simulink model "systemTest_06_24_14_05_13am"  (R2014a)
settings: Solver=ode45  StartTime=0.0  StopTime=100  RelTol=1e-3
values from neighbouring files (symbols this model uses):
  C = [1 0 0 0 0 0;0 0 1 0 0 0;0 0 0 0 1 0]    [parameters1.m]
  friX1 = 4    [initial_parameters.m]    (also in parameters1.m)
  friX2 = 0.76462    [initial_parameters.m]    (also in parameters1.m)
  friY = 8    [initial_parameters.m]    (also in parameters1.m)
  friZ = 4    [initial_parameters.m]    (also in parameters1.m)
  I = 1/12*m*((2*ry1)^2 + (2*rx1)^2)    (= 25.431685482)    [initial_parameters.m]    (also in parameters1.m = 15)
  inputBound = [minInput maxInput]    [parameters1.m]
  K = [1000 1000 1000 10 10 1 1]    [parameters1.m]
  k1m = 50    [parameters1.m]
  k1x = 100    [parameters1.m]
  k1y = 100    [parameters1.m]
  k2m = 25    [parameters1.m]
  k2x = 60    [parameters1.m]
  k2y = 60    [parameters1.m]
  m = 46.27    [initial_parameters.m]    (also in parameters1.m)
  rx1 = -1.2474    [initial_parameters.m]    (also in parameters1.m = -0.7)
  rx2 = rx1    (= -1.2474)    [initial_parameters.m]    (also in parameters1.m = -0.7)
  ry1 = 12*intom    (= 0.3048)    [initial_parameters.m]    (also in parameters1.m)
  ry2 = -12*intom    (= -0.3048)    [initial_parameters.m]    (also in parameters1.m)
libraries: simulink x6
settings Model: Creator=propagator  LastModifiedBy=propagator

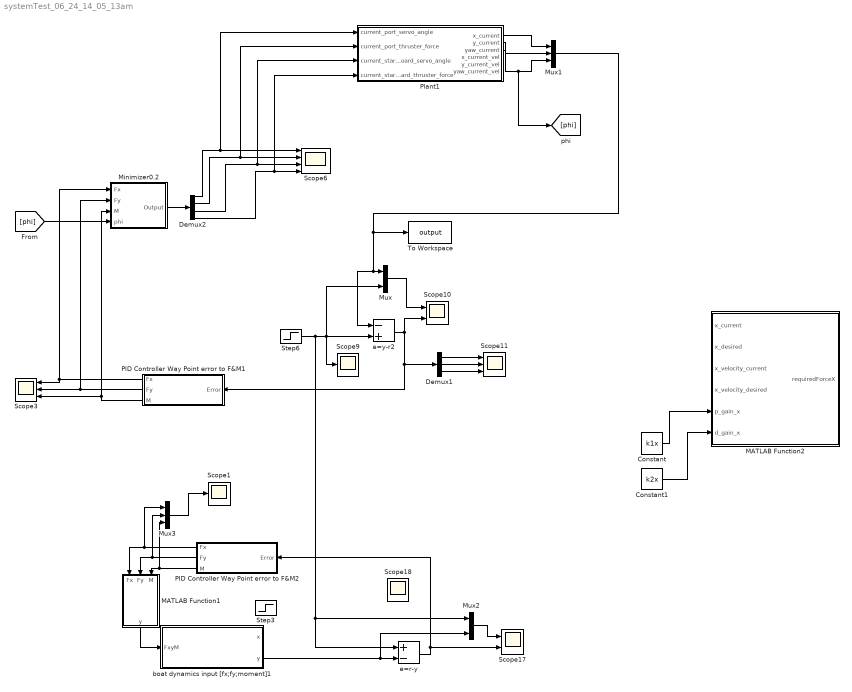
== system systemTest_06_24_14_05_13am ==
  Constant : Constant  Value=k1x
  Constant1 : Constant  Value=k2x
  Demux1 : Demux  Outputs=3
  Demux2 : Demux
  MATLAB Function1 : MATLAB Function  TreatAsAtomicUnit=on
  MATLAB Function2 : MATLAB Function  TreatAsAtomicUnit=on
  Minimizer0.2 : Subsystem  mask{rx1=rx1, rx2=rx2, ry1=ry1, ry2=ry2, C=K, inputBound=inputBound, m=m, I=I}
      mask prompts: C "Performance Gain"; inputBound "Input Bounds"; m "Boat Mass"; I "Boat Inertia"
      mask TypeOptions m: Constant6/Value
      mask TypeOptions I: Constant7/Value
  Mux : Mux  Inputs=2
  Mux1 : Mux  Inputs=3
  Mux2 : Mux  Inputs=2
  Mux3 : Mux  Inputs=3
  PID Controller Way Point error to F&M1 : Subsystem
  PID Controller Way Point error to F&M2 : Subsystem
  Plant1 : Subsystem  mask{rx1=rx1, ry1=ry1, ry2=ry2, M=m, I=I, friX1=friX1, friX2=friX2, friY=friY, friZ=friZ}
      mask TypeOptions rx1: Constant/Value
      mask TypeOptions friX1: Constant1/Value
      mask TypeOptions friX2: Constant8/Value
      mask TypeOptions friY: Constant7/Value
      mask TypeOptions friZ: Constant9/Value
  Scope1 : Scope
      settings: YMin=-0.014  YMax=0  SaveName=ScopeData4
  Scope10 : Scope  NumInputPorts=2
      settings: YMin=0~-0.04  YMax=2~0.025  SaveName=ScopeData9
  Scope11 : Scope  NumInputPorts=3
      settings: YMin=8.65~2.725~-26.6  YMax=8.975~2.925~-25.6  SaveName=ScopeData11
  Scope17 : Scope  NumInputPorts=2
      settings: YMin=0~0  YMax=70~17
  Scope18 : Scope
      settings: SaveName=ScopeData2
  Scope3 : Scope  NumInputPorts=3
      settings: YMin=-1.25~-1~7000  YMax=0.75~1~7000  SaveName=ScopeData3
  Scope6 : Scope  NumInputPorts=4
      settings: YMin=-28~-100~15~0  YMax=-15~0~28~100  SaveName=ScopeData5
  Scope9 : Scope
      settings: SaveName=ScopeData8
  Step3 : Step  Before=[0;0;0]  After=[15;1;1]  SampleTime=0
  Step6 : Step  Before=[0;0;0]  After=[10;0;0]  SampleTime=0
  To Workspace : ToWorkspace  VariableName=output  SaveFormat=Timeseries  SampleTime=-1
  boat dynamics input [fx;fy;moment]1 : Subsystem  mask{M=m, I=I, fw=0, kr=0, C=C}
      mask prompts: M "Mass"; I "Inert"; fw "Water Friction"; kr "Rotational water Friction"; C "Output Matrix"
  e=r-y : Sum  Inputs=+-
  e=y-r2 : Sum  Inputs=-+
  wires:
  Demux2/1 -> Plant1/1(current_port_servo_angle), Scope6/1
  Demux2/2 -> Plant1/2(current_port_thruster_force), Scope6/2
  Demux2/3 -> Plant1/3(current_starboard_servo_angle), Scope6/3
  Demux2/4 -> Plant1/4(current_starboard_thruster_force), Scope6/4
  Minimizer0.2/1(Output) -> Demux2/1
  Step6/1 -> Mux2/1, e=r-y/1, Mux/2, e=y-r2/2, Scope9/1
  e=y-r2/1 -> PID Controller Way Point error to F&M1/1(Error), Demux1/1, Scope10/2
  Mux/1 -> Scope10/1
  PID Controller Way Point error to F&M1/1(Fx) -> Minimizer0.2/1(Fx), Scope3/1
  PID Controller Way Point error to F&M1/2(Fy) -> Scope3/2, Minimizer0.2/2(Fy)
  PID Controller Way Point error to F&M1/3(M) -> Scope3/3, Minimizer0.2/3(M)
  Demux1/3 -> Scope11/3
  Demux1/2 -> Scope11/2
  Demux1/1 -> Scope11/1
  [phi] -> Minimizer0.2/4(phi)
  Plant1/3(yaw_current) -> Mux1/3, [phi]
  Plant1/2(y_current) -> Mux1/2
  Plant1/1(x_current) -> Mux1/1
  Mux1/1 -> e=y-r2/1, Mux/1, To Workspace/1
  e=r-y/1 -> PID Controller Way Point error to F&M2/1(Error), Scope17/2
  PID Controller Way Point error to F&M2/1(Fx) -> Mux3/1, MATLAB Function1/1(Fx)
  MATLAB Function1/1(y) -> boat dynamics input [fx;fy;moment]1/1(FxyM)
  PID Controller Way Point error to F&M2/2(Fy) -> Mux3/2, MATLAB Function1/2(Fy)
  PID Controller Way Point error to F&M2/3(M) -> Mux3/3, MATLAB Function1/3(M)
  boat dynamics input [fx;fy;moment]1/2(y) -> Mux2/2, e=r-y/2
  Mux2/1 -> Scope17/1
  Mux3/1 -> Scope1/1
  Constant1/1 -> MATLAB Function2/6(d_gain_x)
  Constant/1 -> MATLAB Function2/5(p_gain_x)

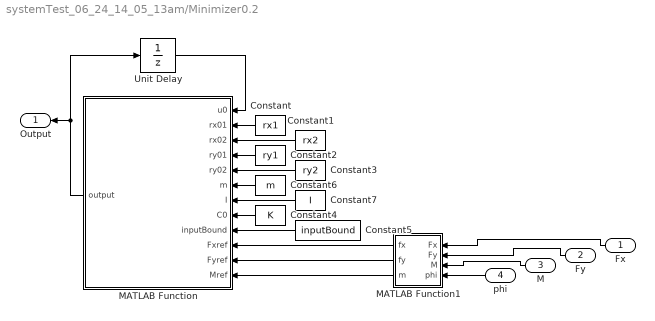
== system systemTest_06_24_14_05_13am/Minimizer0.2 ==
  Fx : Inport
  Fy : Inport  Port=2
  M : Inport  Port=3
  phi : Inport  Port=4
  Constant : Constant  Value=rx1
  Constant1 : Constant  Value=rx2
  Constant2 : Constant  Value=ry1
  Constant3 : Constant  Value=ry2
  Constant4 : Constant  Value=K
  Constant5 : Constant  Value=inputBound
  Constant6 : Constant  Value=m
  Constant7 : Constant  Value=I
  MATLAB Function : MATLAB Function  TreatAsAtomicUnit=on
  MATLAB Function1 : MATLAB Function  TreatAsAtomicUnit=on
  Unit Delay : UnitDelay  InitialCondition=[0;0;0;0]  SampleTime=-1
  Output : Outport
  wires:
  Constant/1 -> MATLAB Function/2(rx01)
  Constant1/1 -> MATLAB Function/3(rx02)
  Constant2/1 -> MATLAB Function/4(ry01)
  Constant4/1 -> MATLAB Function/8(C0)
  Unit Delay/1 -> MATLAB Function/1(u0)
  MATLAB Function/1(output) -> Unit Delay/1, Output/1
  Constant5/1 -> MATLAB Function/9(inputBound)
  Constant3/1 -> MATLAB Function/5(ry02)
  MATLAB Function1/3(m) -> MATLAB Function/12(Mref)
  MATLAB Function1/2(fy) -> MATLAB Function/11(Fyref)
  MATLAB Function1/1(fx) -> MATLAB Function/10(Fxref)
  Fy/1 -> MATLAB Function1/2(Fy)
  Fx/1 -> MATLAB Function1/1(Fx)
  M/1 -> MATLAB Function1/3(M)
  phi/1 -> MATLAB Function1/4(phi)
  Constant6/1 -> MATLAB Function/6(m)
  Constant7/1 -> MATLAB Function/7(I)

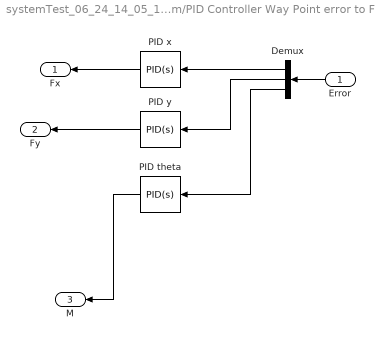
== system systemTest_06_24_14_05_13am/PID Controller Way Point error to F&M1 ==
  Error : Inport
  Demux : Demux  Outputs=3
  PID theta : simulink/Continuous/PID Controller  Controller=PID  TimeDomain=Continuous-time  SampleTime=1  IntegratorMethod=Forward Euler  FilterMethod=Forward Euler  Form=Parallel  P=k1m  I=0  D=k2m  N=3.646824066771  InitialConditionSource=internal  InitialConditionForIntegrator=0  InitialConditionForFilter=0  ExternalReset=none  LimitOutput=off  UpperSaturationLimit=inf  LowerSaturationLimit=-inf  LinearizeAsGain=off  AntiWindupMode=none  Kb=1  TrackingMode=off  Kt=1  PParamMin=[]  PParamMax=[]  IParamMin=[]  IParamMax=[]  DParamMin=[]  DParamMax=[]  NParamMin=[]  NParamMax=[]  KbParamMin=[]  KbParamMax=[]  KtParamMin=[]  KtParamMax=[]  POutMin=[]  POutMax=[]  IOutMin=[]  IOutMax=[]  DOutMin=[]  DOutMax=[]  NOutMin=[]  NOutMax=[]  KbOutMin=[]  KbOutMax=[]  KtOutMin=[]  KtOutMax=[]  IntegratorOutMin=[]  IntegratorOutMax=[]  FilterOutMin=[]  FilterOutMax=[]  SumOutMin=[]  SumOutMax=[]  SumI1OutMin=[]  SumI1OutMax=[]  SumI2OutMin=[]  SumI2OutMax=[]  SumI3OutMin=[]  SumI3OutMax=[]  SumDOutMin=[]  SumDOutMax=[]  SaturationOutMin=[]  SaturationOutMax=[]  IntegratorContinuousStateAttributes=''  IntegratorStateMustResolveToSignalObject=off  IntegratorRTWStateStorageClass=Auto  FilterContinuousStateAttributes=''  FilterStateMustResolveToSignalObject=off  FilterRTWStateStorageClass=Auto
  PID x : simulink/Continuous/PID Controller  Controller=PID  TimeDomain=Continuous-time  SampleTime=1  IntegratorMethod=Forward Euler  FilterMethod=Forward Euler  Form=Parallel  P=k1x  I=0  D=k2x  N=3.646824066771  InitialConditionSource=internal  InitialConditionForIntegrator=0  InitialConditionForFilter=0  ExternalReset=none  LimitOutput=off  UpperSaturationLimit=inf  LowerSaturationLimit=-inf  LinearizeAsGain=off  AntiWindupMode=none  Kb=1  TrackingMode=off  Kt=1  PParamMin=[]  PParamMax=[]  IParamMin=[]  IParamMax=[]  DParamMin=[]  DParamMax=[]  NParamMin=[]  NParamMax=[]  KbParamMin=[]  KbParamMax=[]  KtParamMin=[]  KtParamMax=[]  POutMin=[]  POutMax=[]  IOutMin=[]  IOutMax=[]  DOutMin=[]  DOutMax=[]  NOutMin=[]  NOutMax=[]  KbOutMin=[]  KbOutMax=[]  KtOutMin=[]  KtOutMax=[]  IntegratorOutMin=[]  IntegratorOutMax=[]  FilterOutMin=[]  FilterOutMax=[]  SumOutMin=[]  SumOutMax=[]  SumI1OutMin=[]  SumI1OutMax=[]  SumI2OutMin=[]  SumI2OutMax=[]  SumI3OutMin=[]  SumI3OutMax=[]  SumDOutMin=[]  SumDOutMax=[]  SaturationOutMin=[]  SaturationOutMax=[]  IntegratorContinuousStateAttributes=''  IntegratorStateMustResolveToSignalObject=off  IntegratorRTWStateStorageClass=Auto  FilterContinuousStateAttributes=''  FilterStateMustResolveToSignalObject=off  FilterRTWStateStorageClass=Auto
  PID y : simulink/Continuous/PID Controller  Controller=PID  TimeDomain=Continuous-time  SampleTime=1  IntegratorMethod=Forward Euler  FilterMethod=Forward Euler  Form=Parallel  P=k1y  I=0  D=k2y  N=4  InitialConditionSource=internal  InitialConditionForIntegrator=0  InitialConditionForFilter=0  ExternalReset=none  LimitOutput=off  UpperSaturationLimit=inf  LowerSaturationLimit=-inf  LinearizeAsGain=off  AntiWindupMode=none  Kb=1  TrackingMode=off  Kt=1  PParamMin=[]  PParamMax=[]  IParamMin=[]  IParamMax=[]  DParamMin=[]  DParamMax=[]  NParamMin=[]  NParamMax=[]  KbParamMin=[]  KbParamMax=[]  KtParamMin=[]  KtParamMax=[]  POutMin=[]  POutMax=[]  IOutMin=[]  IOutMax=[]  DOutMin=[]  DOutMax=[]  NOutMin=[]  NOutMax=[]  KbOutMin=[]  KbOutMax=[]  KtOutMin=[]  KtOutMax=[]  IntegratorOutMin=[]  IntegratorOutMax=[]  FilterOutMin=[]  FilterOutMax=[]  SumOutMin=[]  SumOutMax=[]  SumI1OutMin=[]  SumI1OutMax=[]  SumI2OutMin=[]  SumI2OutMax=[]  SumI3OutMin=[]  SumI3OutMax=[]  SumDOutMin=[]  SumDOutMax=[]  SaturationOutMin=[]  SaturationOutMax=[]  IntegratorContinuousStateAttributes=''  IntegratorStateMustResolveToSignalObject=off  IntegratorRTWStateStorageClass=Auto  FilterContinuousStateAttributes=''  FilterStateMustResolveToSignalObject=off  FilterRTWStateStorageClass=Auto
  Fx : Outport
  Fy : Outport  Port=2
  M : Outport  Port=3
  wires:
  Demux/1 -> PID x/1
  Demux/2 -> PID y/1
  Demux/3 -> PID theta/1
  Error/1 -> Demux/1
  PID y/1 -> Fy/1
  PID x/1 -> Fx/1
  PID theta/1 -> M/1

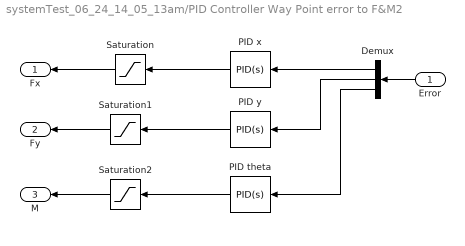
== system systemTest_06_24_14_05_13am/PID Controller Way Point error to F&M2 ==
  Error : Inport
  Demux : Demux  Outputs=3
  PID theta : simulink/Continuous/PID Controller  Controller=PID  TimeDomain=Continuous-time  SampleTime=1  IntegratorMethod=Forward Euler  FilterMethod=Forward Euler  Form=Parallel  P=k1m  I=0  D=k2m  N=3.646824066771  InitialConditionSource=internal  InitialConditionForIntegrator=0  InitialConditionForFilter=0  ExternalReset=none  LimitOutput=off  UpperSaturationLimit=inf  LowerSaturationLimit=-inf  LinearizeAsGain=off  AntiWindupMode=none  Kb=1  TrackingMode=off  Kt=1  PParamMin=[]  PParamMax=[]  IParamMin=[]  IParamMax=[]  DParamMin=[]  DParamMax=[]  NParamMin=[]  NParamMax=[]  KbParamMin=[]  KbParamMax=[]  KtParamMin=[]  KtParamMax=[]  POutMin=[]  POutMax=[]  IOutMin=[]  IOutMax=[]  DOutMin=[]  DOutMax=[]  NOutMin=[]  NOutMax=[]  KbOutMin=[]  KbOutMax=[]  KtOutMin=[]  KtOutMax=[]  IntegratorOutMin=[]  IntegratorOutMax=[]  FilterOutMin=[]  FilterOutMax=[]  SumOutMin=[]  SumOutMax=[]  SumI1OutMin=[]  SumI1OutMax=[]  SumI2OutMin=[]  SumI2OutMax=[]  SumI3OutMin=[]  SumI3OutMax=[]  SumDOutMin=[]  SumDOutMax=[]  SaturationOutMin=[]  SaturationOutMax=[]  IntegratorContinuousStateAttributes=''  IntegratorStateMustResolveToSignalObject=off  IntegratorRTWStateStorageClass=Auto  FilterContinuousStateAttributes=''  FilterStateMustResolveToSignalObject=off  FilterRTWStateStorageClass=Auto
  PID x : simulink/Continuous/PID Controller  Controller=PID  TimeDomain=Continuous-time  SampleTime=1  IntegratorMethod=Forward Euler  FilterMethod=Forward Euler  Form=Parallel  P=k1x  I=0  D=k2x  N=3.646824066771  InitialConditionSource=internal  InitialConditionForIntegrator=0  InitialConditionForFilter=0  ExternalReset=none  LimitOutput=off  UpperSaturationLimit=inf  LowerSaturationLimit=-inf  LinearizeAsGain=off  AntiWindupMode=none  Kb=1  TrackingMode=off  Kt=1  PParamMin=[]  PParamMax=[]  IParamMin=[]  IParamMax=[]  DParamMin=[]  DParamMax=[]  NParamMin=[]  NParamMax=[]  KbParamMin=[]  KbParamMax=[]  KtParamMin=[]  KtParamMax=[]  POutMin=[]  POutMax=[]  IOutMin=[]  IOutMax=[]  DOutMin=[]  DOutMax=[]  NOutMin=[]  NOutMax=[]  KbOutMin=[]  KbOutMax=[]  KtOutMin=[]  KtOutMax=[]  IntegratorOutMin=[]  IntegratorOutMax=[]  FilterOutMin=[]  FilterOutMax=[]  SumOutMin=[]  SumOutMax=[]  SumI1OutMin=[]  SumI1OutMax=[]  SumI2OutMin=[]  SumI2OutMax=[]  SumI3OutMin=[]  SumI3OutMax=[]  SumDOutMin=[]  SumDOutMax=[]  SaturationOutMin=[]  SaturationOutMax=[]  IntegratorContinuousStateAttributes=''  IntegratorStateMustResolveToSignalObject=off  IntegratorRTWStateStorageClass=Auto  FilterContinuousStateAttributes=''  FilterStateMustResolveToSignalObject=off  FilterRTWStateStorageClass=Auto
  PID y : simulink/Continuous/PID Controller  Controller=PID  TimeDomain=Continuous-time  SampleTime=1  IntegratorMethod=Forward Euler  FilterMethod=Forward Euler  Form=Parallel  P=k1y  I=0  D=k2y  N=4  InitialConditionSource=internal  InitialConditionForIntegrator=0  InitialConditionForFilter=0  ExternalReset=none  LimitOutput=off  UpperSaturationLimit=inf  LowerSaturationLimit=-inf  LinearizeAsGain=off  AntiWindupMode=none  Kb=1  TrackingMode=off  Kt=1  PParamMin=[]  PParamMax=[]  IParamMin=[]  IParamMax=[]  DParamMin=[]  DParamMax=[]  NParamMin=[]  NParamMax=[]  KbParamMin=[]  KbParamMax=[]  KtParamMin=[]  KtParamMax=[]  POutMin=[]  POutMax=[]  IOutMin=[]  IOutMax=[]  DOutMin=[]  DOutMax=[]  NOutMin=[]  NOutMax=[]  KbOutMin=[]  KbOutMax=[]  KtOutMin=[]  KtOutMax=[]  IntegratorOutMin=[]  IntegratorOutMax=[]  FilterOutMin=[]  FilterOutMax=[]  SumOutMin=[]  SumOutMax=[]  SumI1OutMin=[]  SumI1OutMax=[]  SumI2OutMin=[]  SumI2OutMax=[]  SumI3OutMin=[]  SumI3OutMax=[]  SumDOutMin=[]  SumDOutMax=[]  SaturationOutMin=[]  SaturationOutMax=[]  IntegratorContinuousStateAttributes=''  IntegratorStateMustResolveToSignalObject=off  IntegratorRTWStateStorageClass=Auto  FilterContinuousStateAttributes=''  FilterStateMustResolveToSignalObject=off  FilterRTWStateStorageClass=Auto
  Saturation : Saturate  UpperLimit=100  LowerLimit=-100
  Saturation1 : Saturate  UpperLimit=100  LowerLimit=-100
  Saturation2 : Saturate  UpperLimit=50  LowerLimit=-50
  Fx : Outport
  Fy : Outport  Port=2
  M : Outport  Port=3
  wires:
  Demux/1 -> PID x/1
  Demux/2 -> PID y/1
  Demux/3 -> PID theta/1
  Error/1 -> Demux/1
  PID x/1 -> Saturation/1
  Saturation/1 -> Fx/1
  PID y/1 -> Saturation1/1
  Saturation1/1 -> Fy/1
  PID theta/1 -> Saturation2/1
  Saturation2/1 -> M/1

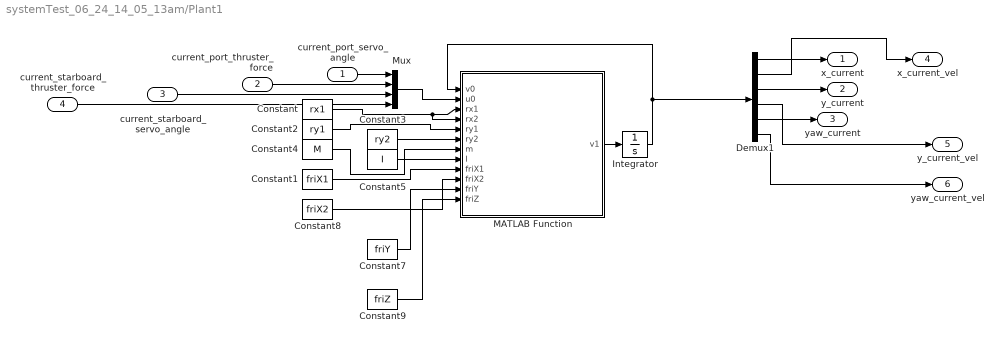
== system systemTest_06_24_14_05_13am/Plant1 ==
  current_port_servo_angle : Inport
  current_port_thruster_force : Inport  Port=2
  current_starboard_servo_angle : Inport  Port=3
  current_starboard_thruster_force : Inport  Port=4
  Constant : Constant  Value=rx1
  Constant1 : Constant  Value=friX1
  Constant2 : Constant  Value=ry1
  Constant3 : Constant  Value=ry2
  Constant4 : Constant  Value=M
  Constant5 : Constant  Value=I
  Constant7 : Constant  Value=friY
  Constant8 : Constant  Value=friX2
  Constant9 : Constant  Value=friZ
  Demux1 : Demux  Outputs=6
  Integrator : Integrator  InitialCondition=[0 0 0 0 0 0]
  MATLAB Function : MATLAB Function  TreatAsAtomicUnit=on
  Mux : Mux
  x_current : Outport
  y_current : Outport  Port=2
  yaw_current : Outport  Port=3
  x_current_vel : Outport  Port=4
  y_current_vel : Outport  Port=5
  yaw_current_vel : Outport  Port=6
  wires:
  Constant/1 -> MATLAB Function/3(rx1), MATLAB Function/4(rx2)
  Constant2/1 -> MATLAB Function/5(ry1)
  Constant3/1 -> MATLAB Function/6(ry2)
  Constant4/1 -> MATLAB Function/7(m)
  Constant5/1 -> MATLAB Function/8(I)
  MATLAB Function/1(v1) -> Integrator/1
  Integrator/1 -> MATLAB Function/1(v0), Demux1/1
  current_port_servo_angle/1 -> Mux/1
  current_port_thruster_force/1 -> Mux/2
  current_starboard_servo_angle/1 -> Mux/3
  current_starboard_thruster_force/1 -> Mux/4
  Mux/1 -> MATLAB Function/2(u0)
  Constant1/1 -> MATLAB Function/9(friX1)
  Constant7/1 -> MATLAB Function/11(friY)
  Constant9/1 -> MATLAB Function/12(friZ)
  Constant8/1 -> MATLAB Function/10(friX2)
  Demux1/5 -> yaw_current/1
  Demux1/3 -> y_current/1
  Demux1/1 -> x_current/1
  Demux1/2 -> x_current_vel/1
  Demux1/4 -> y_current_vel/1
  Demux1/6 -> yaw_current_vel/1

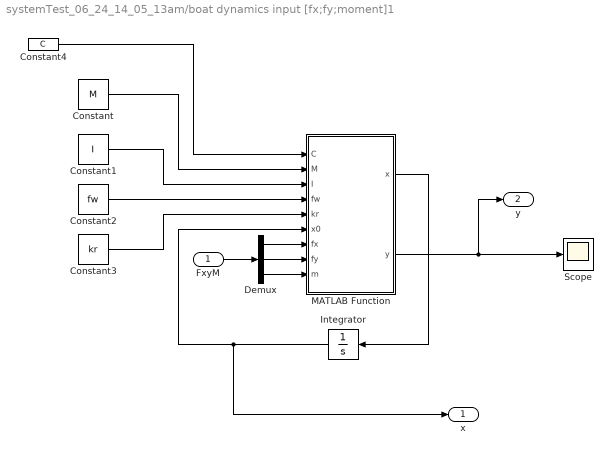
== system systemTest_06_24_14_05_13am/boat dynamics input [fx;fy;moment]1 ==
  FxyM : Inport
  Constant : Constant  Value=M
  Constant1 : Constant  Value=I
  Constant2 : Constant  Value=fw
  Constant3 : Constant  Value=kr
  Constant4 : Constant  Value=C
  Demux : Demux  Outputs=3
  Integrator : Integrator  InitialCondition=[0 0 0 0 0 0]
  MATLAB Function : MATLAB Function  TreatAsAtomicUnit=on
  Scope : Scope
  x : Outport
  y : Outport  Port=2
  wires:
  MATLAB Function/2(y) -> Scope/1, y/1
  Integrator/1 -> x/1, MATLAB Function/6(x0)
  Constant/1 -> MATLAB Function/2(M)
  Constant1/1 -> MATLAB Function/3(I)
  Constant2/1 -> MATLAB Function/4(fw)
  Constant3/1 -> MATLAB Function/5(kr)
  Constant4/1 -> MATLAB Function/1(C)
  MATLAB Function/1(x) -> Integrator/1
  FxyM/1 -> Demux/1
  Demux/1 -> MATLAB Function/7(fx)
  Demux/2 -> MATLAB Function/8(fy)
  Demux/3 -> MATLAB Function/9(m)

== matlab function systemTest_06_24_14_05_13am/MATLAB Function2 ==
  data: x_current input; requiredForceX output; x_desired input; x_velocity_current input; x_velocity_desired input; p_gain_x input; d_gain_x input
function requiredForceX = fcn(x_current,x_desired,x_velocity_current,x_velocity_desired, p_gain_x, d_gain_x)
%#codegen


requiredForceX = p_gain_x * (x_desired - x_current) + d_gain_x * (x_velocity_desired - x_velocity_current);
end

== matlab function systemTest_06_24_14_05_13am/Plant1/MATLAB Function ==
  data: v0 input; v1 output; u0 input; rx1 input; rx2 input; ry1 input; ry2 input; m input; I input; friX1 input; friX2 input; friY input; friZ input

function v1   = boatDynamics(v0, u0, rx1, rx2, ry1, ry2, m, I, friX1,friX2, friY, friZ)

    % %%%%%%%%%%%%%%%%%%%%%%%%%%%%%%%%%%%%%%%%%%%% %
    %    v = [x...          %    u = [theta1...    %
    %        x_dot...       %        f1...         %
    %        y...           %        theta2...     %
    %        y_dot...       %        f2]           %
    %        theta...       %                      %
    %        theta_dot];    %                      %
    % %%%%%%%%%%%%%%%%%%%%%%%%%%%%%%%%%%%%%%%%%%%% %
    
    v11 = v0(2);
    v12 = u0(2)/m*cosd(u0(1)+v0(5)) + u0(4)/m*cosd(u0(3)+v0(5)) - (friX1*v0(2)*(cosd(v0(5))+sind(v0(5))) - friX2*(v0(2)*(cosd(v0(5))+sind(v0(5))))^2);
    v13 = v0(4);
    v14 = u0(2)/m*sind(u0(1)+v0(5)) + u0(4)/m*sind(u0(3)+v0(5)) - friY*v0(4)*(-sind(v0(5))+cosd(v0(5)));
    v15 = v0(6);
    v16 = -rx1/I*u0(2)*sind(u0(1)) + ry1/I*u0(2)*cosd(u0(1)) - rx2/I*u0(4)*sind(u0(3)) + ry2/I*u0(4)*cosd(u0(3)) - friZ*v0(6);
   
    v1 = [v11;v12;v13;v14;v15;v16];
    
end

== matlab function systemTest_06_24_14_05_13am/Minimizer0.2/MATLAB Function ==
  data: u0 input; output output; rx01 input; rx02 input; ry01 input; ry02 input; m input; I input; C0 input; inputBound input; Fxref input; Fyref input; Mref input
function output = Minimizer(u0, rx01, rx02, ry01, ry02, m, I, C0, inputBound, Fxref, Fyref, Mref)

rx1 = rx01; rx2 = rx02;
ry1 = ry01; ry2 = ry02;

C = C0;

%Fxref = Fx; Fyref = Fy; Mref  = M;

gridNum = 10;

grid = boundGrid(inputBound, gridNum, rx1,ry1);

u1 = getMinFromGrid(grid, u0, Fxref, Fyref, Mref, rx1, rx2, ry1, ry2, C, m, I);

% u1 = u0;

% %     for k = 1:20
% %         h = getDirection(u1, u0, Fxref, Fyref, Mref, rx1, rx2, ry1, ry2, C);
% %         alpha = getStepSize(u1, u0, h, Fxref, Fyref, Mref, rx1, rx2, ry1, ry2, C);
% %         u1 = u1 + alpha*h;
% %         u1 = checkInputBound(u1,inputBound);
% %     end
    
    output = u1;

end

function output = getMinFromGrid(grid, preinput, Fxref, Fyref, Mref, rx1, rx2, ry1, ry2, C, m, I)

[ii, iii] = size(grid);
v0 = costFunction(grid(1,:), preinput, Fxref, Fyref, Mref, rx1, rx2, ry1, ry2, C, m, I);

output = [grid(1,1);grid(1,2);grid(1,3);grid(1,4)];

for i = 1:ii
    for j = 1:ii
        for k = 1:ii
            for l = 1:ii
                input = [grid(i,1);grid(j,2);grid(k,3);grid(l,4)];
                v1 = costFunction(input,preinput, Fxref, Fyref, Mref, rx1, rx2, ry1, ry2, C, m, I);
                if v0 > v1
                    v0 = v1;
                    output = input;
                else
                end
            end
        end
    end
end

end

function output = checkInputBound(input,inputBound)
k = [0;0;0;0];
    for i = 1:length(input)
        k(i) = sat(input(i),inputBound(i,:));
    end
    output = k;
end

function output = boundGrid(inputBound, gridNum, rx1,ry1)

p = gridNum;

theta1 =    linspace(inputBound(1,1),inputBound(1,2),p)';
f1 =        linspace(inputBound(2,1),inputBound(2,2),p)';
theta2 =    linspace(inputBound(3,1),inputBound(3,2),p)';
f2 =        linspace(inputBound(4,1),inputBound(4,2),p)';

%i = atan(rx1/ry1)*180/pi;

output = [theta1, f1, theta2, f2;...
          inputBound(1,1),  0,      inputBound(3,1),  0;...
             0,    100,    0,    100;...%];
             0,   -100,    0,   -100]; %...
%             i,    0,    i,    0];

end

function output = sat(input, bound)

    if input < bound(1)
        output = bound(1);
    elseif input > bound(2)
        output = bound(2);
    else
        output = input;
    end

end

function output = getStepSize(input, preinput, h, Fxref, Fyref, Mref, rx1, rx2, ry1, ry2, C, m, I)

    alpha = .001;
    
    u0 = input;
    u1 = input + alpha*h;
    
    v0 = costFunction( u0, preinput, Fxref, Fyref, Mref, rx1, rx2, ry1, ry2, C, m, I );
    v1 = costFunction( u1, preinput, Fxref, Fyref, Mref, rx1, rx2, ry1, ry2, C, m, I);

    while v1 <= v0 && v1 ~= 0
        alpha = alpha + .001;
        u1 = input + alpha*h;
        v0 = v1;
        v1 = costFunction( u1, preinput, Fxref, Fyref, Mref, rx1, rx2, ry1, ry2, C, m, I );
    end
    
    v0 = v1;
    alpha = .0015;

    while v1 <= v0  && v1 ~= 0
        alpha = alpha - 0.0001;
        u1 = input + alpha*h;
        v0 = v1;
        v1 = costFunction( u1, preinput, Fxref, Fyref, Mref, rx1, rx2, ry1, ry2, C, m, I );
    end


    output = alpha;

end

function output = costFunction(input, preinput, Fxref, Fyref, Mref, rx1, rx2, ry1, ry2, C, m, I)

    theta1  = input(1);
    f1      = input(2);
    theta2  = input(3);
    f2      = input(4);
    
    pretheta1   = preinput(1);
    pretheta2   = preinput(3);

    Fx = (f1*cosd(theta1) + f2*cosd(theta2))/m;
    Fy = (f1*sind(theta1) + f2*sind(theta2))/m;
    M = (-rx1*f1*sind(theta1) + ry1*f1*cosd(theta1) - rx2*f2*sind(theta2)...
        + ry2*f2*cosd(theta2))/I;

    output = C(1)*(Fx-Fxref)^2 +...
        C(2)*(Fy-Fyref)^2 +...
        C(3)*(M-Mref)^2  +...
        C(4)*f1^2 +...
        C(5)*f2^2 +...
        C(6)*(theta1 - pretheta1)^2 +...
        C(7)*(theta2 - pretheta2)^2;% +...
%         C(5)*theta1^2 +...
%         C(5)*theta2^2;

end

function output = getDirection(input, preinput, Fxref, Fyref, Mref, rx1, rx2, ry1, ry2, C, m, I)

hsd = SteepestDescent(input, preinput, Fxref, Fyref, Mref, rx1, rx2, ry1, ry2, C, m, I);

output = zeros(4,1);

    for i = 1:length(hsd)
        output(i) = hsd(i);
    end
    
end

function output = SteepestDescent(input, preinput, Fxref, Fyref, Mref, rx1, rx2, ry1, ry2, C, m, I)

theta1  = input(1);
f1      = input(2);
theta2  = input(3);
f2      = input(4);

pretheta1   = preinput(1);
pretheta2   = preinput(3);

dVdtheta1 = C(3)*(f1*ry1*cosd(theta1)...
    - f1*rx1*sind(theta1))*(f1*rx1*cosd(theta1)...
    - Mref + f2*rx2*cosd(theta2) + f1*ry1*sin(theta1)...
    + f2*ry2*sind(theta2)) - C(6)*(pretheta1 - theta1)...
    - C(2)*f1*sind(theta1)*(f1*cosd(theta1) - Fyref + f2*cosd(theta2))...
    + C(1)*f1*cosd(theta1)*(Fxref + f1*sind(theta1) + f2*sind(theta2));

dVdf1 = C(4)*f1 + C(1)*sind(theta1)*(Fxref + f1*sin(theta1)...
    + f2*sind(theta2)) + C(2)*cosd(theta1)*(f1*cosd(theta1) - Fyref...
    + f2*cosd(theta2)) + C(3)*(rx1*cosd(theta1)...
    + ry1*sind(theta1))*(f1*rx1*cosd(theta1) - Mref + f2*rx2*cosd(theta2)...
    + f1*ry1*sind(theta1) + f2*ry2*sind(theta2));

dVdtheta2 = C(3)*(f2*ry2*cosd(theta2)...
    - f2*rx2*sind(theta2))*(f1*rx1*cosd(theta1)...
    - Mref + f2*rx2*cosd(theta2) + f1*ry1*sind(theta1)...
    + f2*ry2*sind(theta2)) - C(7)*(pretheta2 - theta2)...
    - C(2)*f2*sind(theta2)*(f1*cosd(theta1) - Fyref + f2*cosd(theta2))...
    + C(1)*f2*cosd(theta2)*(Fxref + f1*sind(theta1) + f2*sind(theta2));

dVdf2 = C(5)*f2 + C(1)*sind(theta2)*(Fxref + f1*sind(theta1)...
    + f2*sind(theta2)) + C(2)*cosd(theta2)*(f1*cosd(theta1) - Fyref...
    + f2*cosd(theta2)) + C(3)*(rx2*cosd(theta2)...
    + ry2*sind(theta2))*(f1*rx1*cosd(theta1) - Mref + f2*rx2*cosd(theta2)...
    + f1*ry1*sind(theta1) + f2*ry2*sind(theta2));
 
output = -[dVdtheta1; dVdf1; dVdtheta2; dVdf2];

end

== matlab function systemTest_06_24_14_05_13am/Minimizer0.2/MATLAB Function1 ==
  data: Fx input; fx output; Fy input; M input; fy output; m output; phi input
function [fx,fy,m] = fcn(Fx,Fy,M, phi)
%#codegen

R = [cosd(phi) -sind(phi) 0;...
        sind(phi)  cosd(phi) 0;...
        0           0       1];
    
    FxyM = R'*[Fx;Fy;M];
    
    fx = FxyM(1);
    fy = FxyM(2);
    m = FxyM(3);
    
end

== matlab function systemTest_06_24_14_05_13am/MATLAB Function1 ==
  data: Fx input; y output; Fy input; M input
function y = fcn(Fx,Fy,M)
%#codegen

y = [Fx;Fy;M];

== matlab function systemTest_06_24_14_05_13am/boat dynamics input [fx;fy;moment]1/MATLAB Function ==
  data: C input; x output; M input; I input; fw input; kr input; x0 input; fx input; y output; fy input; m input
function [x,y] = systemstep(C,M,I,fw,kr,x0,fx,fy,m)

   % status vector y=[x;x_dot;y;_y_dot;theta;theta_dot]
   % forces u=[fx;fy;m]
   % contant parameters {mass; rotational inertia; friction coefficients }
   
   x1 = x0(2);
   x2 = fx/M - 0*x0(2)*fw;
   x3 = x0(4);
   x4 = fy/M - 0*x0(4)*fw;
   x5 = x0(6);
   x6 = m/I - 0*x0(6)*kr;

   x=[x1;x2;x3;x4;x5;x6];
   
   y = C*x0;
